simulink model "Funtional_architecture"  (R2023b)
settings: Solver=VariableStepAuto  StartTime=0.0  StopTime=10.0  RelTol=1e-3
settings Model: Creator=Cristian  LastModifiedBy=Cristian

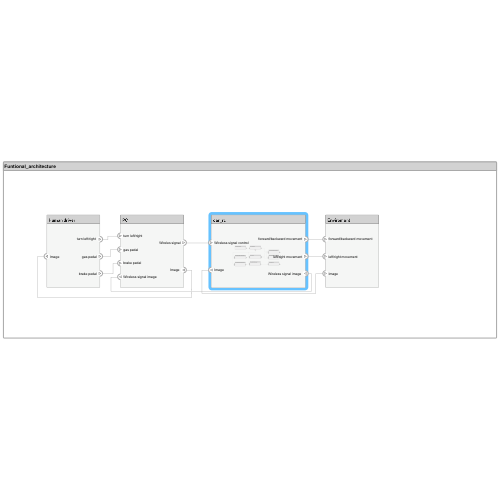
[thumbnail: Simulink's stored preview of the top-level diagram]
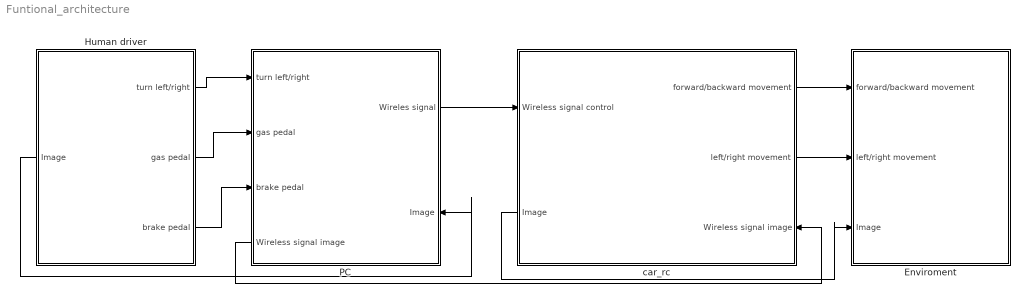
== system Funtional_architecture ==
  Enviroment : Subsystem
      settings: PortSchema="{\"entries\":[{\"content\":{\"headerSize\":26,\"margin\":15,\"minimumSpacing\":25,\"sides\":[{\"content\":{\"connectorIds\":[\"In1\",\"In3\",\"In2\"]},\"type\":\"ConnectorPlacement.EquallySpacedRectSide\",\"uuid\":\"91bad662-27d1-4d59-a5f7-74e6234eecbb\"},{\"content\":{\"side\":\"RIGHT\"},\"type\":\"ConnectorPlacement.EquallySpacedRectSide\",\"uuid\":\"82f07ea1-3832-41bc-8b24-b125feaa4e94\"},{\"content\":{\"side\":\"TOP\"},\"type\":\"ConnectorPlacement.EquallySpacedRectSide\",\"uuid\":\"b3c061be-027d-4d14-becf-7da3730053c6\"}]},\"type\":\"ConnectorPlacement.EquallySpacedConnector\",\"uuid\":\"02efdf8c-4bde-4c3a-95c2-4e1e7b2b6121\"}],\"packageUris\":[\"http://schema.mathworks.com/mf0/Connector/R2020b\"],\"version\":\"1.0\"}"
  Human driver : Subsystem
      settings: PortSchema="{\"entries\":[{\"content\":{\"headerSize\":26,\"margin\":15,\"minimumSpacing\":25,\"sides\":[{\"content\":{\"connectorIds\":[\"Out4\"]},\"type\":\"ConnectorPlacement.EquallySpacedRectSide\",\"uuid\":\"91bad662-27d1-4d59-a5f7-74e6234eecbb\"},{\"content\":{\"connectorIds\":[\"Out1\",\"Out2\",\"Out3\"],\"side\":\"RIGHT\"},\"type\":\"ConnectorPlacement.EquallySpacedRectSide\",\"uuid\":\"82f07ea1-3832-41bc-8b24-b125feaa4e94\"},{\"content\":{\"side\":\"TOP\"},\"type\":\"ConnectorPlacement.EquallySpacedRectSide\",\"uuid\":\"b3c061be-027d-4d14-becf-7da3730053c6\"}]},\"type\":\"ConnectorPlacement.EquallySpacedConnector\",\"uuid\":\"02efdf8c-4bde-4c3a-95c2-4e1e7b2b6121\"}],\"packageUris\":[\"http://schema.mathworks.com/mf0/Connector/R2020b\"],\"version\":\"1.0\"}"
  PC : Subsystem
      settings: PortSchema="{\"entries\":[{\"content\":{\"headerSize\":26,\"margin\":15,\"minimumSpacing\":25,\"sides\":[{\"content\":{\"connectorIds\":[\"In1\",\"In2\",\"In3\",\"Out2\"]},\"type\":\"ConnectorPlacement.EquallySpacedRectSide\",\"uuid\":\"91bad662-27d1-4d59-a5f7-74e6234eecbb\"},{\"content\":{\"connectorIds\":[\"Out1\",\"In4\"],\"side\":\"RIGHT\"},\"type\":\"ConnectorPlacement.EquallySpacedRectSide\",\"uuid\":\"82f07ea1-3832-41bc-8b24-b125feaa4e94\"},{\"content\":{\"side\":\"TOP\"},\"type\":\"ConnectorPlacement.EquallySpacedRectSide\",\"uuid\":\"b3c061be-027d-4d14-becf-7da3730053c6\"}]},\"type\":\"ConnectorPlacement.EquallySpacedConnector\",\"uuid\":\"02efdf8c-4bde-4c3a-95c2-4e1e7b2b6121\"}],\"packageUris\":[\"http://schema.mathworks.com/mf0/Connector/R2020b\"],\"version\":\"1.0\"}"
  car_rc : Subsystem
      settings: PortSchema="{\"entries\":[{\"content\":{\"headerSize\":26,\"margin\":15,\"minimumSpacing\":25,\"sides\":[{\"content\":{\"connectorIds\":[\"In1\",\"Out2\"]},\"type\":\"ConnectorPlacement.EquallySpacedRectSide\",\"uuid\":\"91bad662-27d1-4d59-a5f7-74e6234eecbb\"},{\"content\":{\"connectorIds\":[\"Out1\",\"Out3\",\"In2\"],\"side\":\"RIGHT\"},\"type\":\"ConnectorPlacement.EquallySpacedRectSide\",\"uuid\":\"82f07ea1-3832-41bc-8b24-b125feaa4e94\"},{\"content\":{\"side\":\"TOP\"},\"type\":\"ConnectorPlacement.EquallySpacedRectSide\",\"uuid\":\"b3c061be-027d-4d14-becf-7da3730053c6\"}]},\"type\":\"ConnectorPlacement.EquallySpacedConnector\",\"uuid\":\"02efdf8c-4bde-4c3a-95c2-4e1e7b2b6121\"}],\"packageUris\":[\"http://schema.mathworks.com/mf0/Connector/R2020b\"],\"version\":\"1.0\"}"
  wires:
  PC/2("Wireless signal image ") -> car_rc/2("Wireless signal image ")
  Human driver/4("Image ") -> PC/4("Image ")
  car_rc/2(Image) -> Enviroment/2(Image)
  Human driver/3(brake pedal) -> PC/3(brake pedal)
  PC/1(Wireles signal) -> car_rc/1(Wireless signal control)
  car_rc/3(left/right movement) -> Enviroment/3(left/right movement)
  car_rc/1(forward/backward movement) -> Enviroment/1(forward/backward movement)
  Human driver/1("turn left/right ") -> PC/1("turn left/right ")
  Human driver/2(gas pedal) -> PC/2(gas pedal)

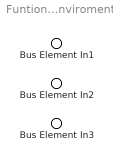
== system Funtional_architecture/Enviroment ==
  Bus Element In1 : Inport  PortName=forward/backward movement
  Bus Element In2 : Inport  Port=2  PortName=Image
  Bus Element In3 : Inport  Port=3  PortName=left/right movement

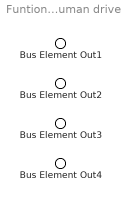
== system Funtional_architecture/Human driver ==
  Bus Element Out1 : Outport  PortName=turn left/right
  Bus Element Out2 : Outport  Port=2  PortName=gas pedal
  Bus Element Out3 : Outport  Port=3  PortName=brake pedal
  Bus Element Out4 : Outport  Port=4  PortName=Image

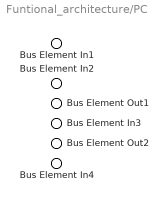
== system Funtional_architecture/PC ==
  Bus Element In1 : Inport  PortName=turn left/right
  Bus Element In2 : Inport  Port=2  PortName=gas pedal
  Bus Element In3 : Inport  Port=3  PortName=brake pedal
  Bus Element In4 : Inport  Port=4  PortName=Image
  Bus Element Out1 : Outport  PortName=Wireles signal
  Bus Element Out2 : Outport  Port=2  PortName=Wireless signal image

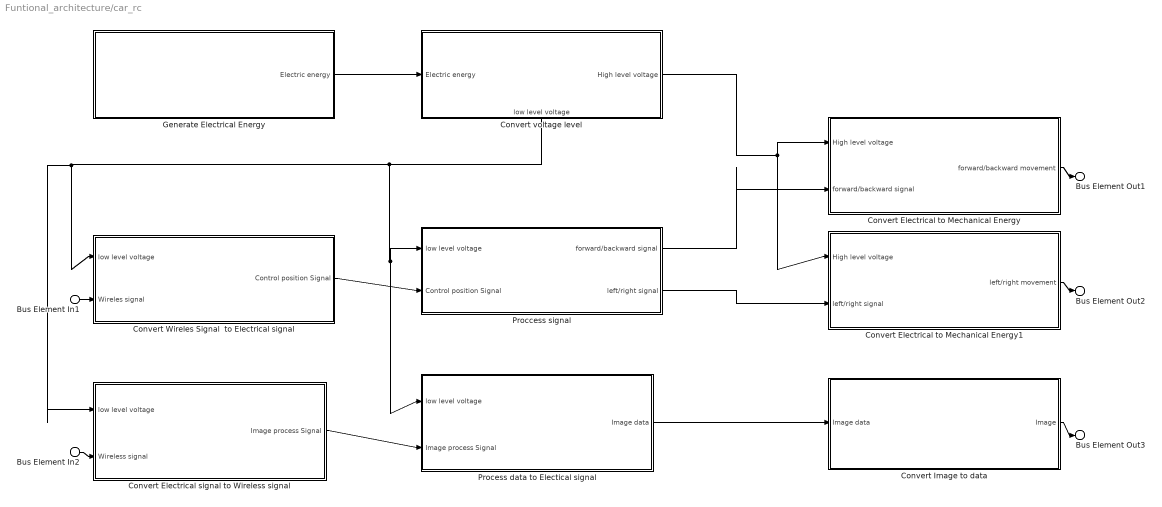
== system Funtional_architecture/car_rc ==
  Bus Element In1 : Inport  PortName=Wireless signal control
  Bus Element In2 : Inport  Port=2  PortName=Wireless signal image
  Convert Electrical signal to Wireless signal : Subsystem
      settings: PortSchema="{\"entries\":[{\"content\":{\"headerSize\":26,\"margin\":15,\"minimumSpacing\":25,\"sides\":[{\"content\":{\"connectorIds\":[\"In1\",\"In2\"]},\"type\":\"ConnectorPlacement.EquallySpacedRectSide\",\"uuid\":\"91bad662-27d1-4d59-a5f7-74e6234eecbb\"},{\"content\":{\"connectorIds\":[\"Out1\"],\"side\":\"RIGHT\"},\"type\":\"ConnectorPlacement.EquallySpacedRectSide\",\"uuid\":\"82f07ea1-3832-41bc-8b24-b125feaa4e94\"},{\"content\":{\"side\":\"TOP\"},\"type\":\"ConnectorPlacement.EquallySpacedRectSide\",\"uuid\":\"b3c061be-027d-4d14-becf-7da3730053c6\"}]},\"type\":\"ConnectorPlacement.EquallySpacedConnector\",\"uuid\":\"02efdf8c-4bde-4c3a-95c2-4e1e7b2b6121\"}],\"packageUris\":[\"http://schema.mathworks.com/mf0/Connector/R2020b\"],\"version\":\"1.0\"}"
  Convert Electrical to Mechanical Energy : Subsystem
      settings: PortSchema="{\"entries\":[{\"content\":{\"headerSize\":26,\"margin\":15,\"minimumSpacing\":25,\"sides\":[{\"content\":{\"connectorIds\":[\"In1\",\"In2\"]},\"type\":\"ConnectorPlacement.EquallySpacedRectSide\",\"uuid\":\"91bad662-27d1-4d59-a5f7-74e6234eecbb\"},{\"content\":{\"connectorIds\":[\"Out1\"],\"side\":\"RIGHT\"},\"type\":\"ConnectorPlacement.EquallySpacedRectSide\",\"uuid\":\"82f07ea1-3832-41bc-8b24-b125feaa4e94\"},{\"content\":{\"side\":\"TOP\"},\"type\":\"ConnectorPlacement.EquallySpacedRectSide\",\"uuid\":\"b3c061be-027d-4d14-becf-7da3730053c6\"}]},\"type\":\"ConnectorPlacement.EquallySpacedConnector\",\"uuid\":\"02efdf8c-4bde-4c3a-95c2-4e1e7b2b6121\"}],\"packageUris\":[\"http://schema.mathworks.com/mf0/Connector/R2020b\"],\"version\":\"1.0\"}"
  Convert Electrical to Mechanical Energy1 : Subsystem
      settings: PortSchema="{\"entries\":[{\"content\":{\"headerSize\":26,\"margin\":15,\"minimumSpacing\":25,\"sides\":[{\"content\":{\"connectorIds\":[\"In1\",\"In2\"]},\"type\":\"ConnectorPlacement.EquallySpacedRectSide\",\"uuid\":\"91bad662-27d1-4d59-a5f7-74e6234eecbb\"},{\"content\":{\"connectorIds\":[\"Out1\"],\"side\":\"RIGHT\"},\"type\":\"ConnectorPlacement.EquallySpacedRectSide\",\"uuid\":\"82f07ea1-3832-41bc-8b24-b125feaa4e94\"},{\"content\":{\"side\":\"TOP\"},\"type\":\"ConnectorPlacement.EquallySpacedRectSide\",\"uuid\":\"b3c061be-027d-4d14-becf-7da3730053c6\"}]},\"type\":\"ConnectorPlacement.EquallySpacedConnector\",\"uuid\":\"02efdf8c-4bde-4c3a-95c2-4e1e7b2b6121\"}],\"packageUris\":[\"http://schema.mathworks.com/mf0/Connector/R2020b\"],\"version\":\"1.0\"}"
  Convert Image to data : Subsystem
      settings: PortSchema="{\"entries\":[{\"content\":{\"headerSize\":26,\"margin\":15,\"minimumSpacing\":25,\"sides\":[{\"content\":{\"connectorIds\":[\"In1\"]},\"type\":\"ConnectorPlacement.EquallySpacedRectSide\",\"uuid\":\"91bad662-27d1-4d59-a5f7-74e6234eecbb\"},{\"content\":{\"connectorIds\":[\"Out1\"],\"side\":\"RIGHT\"},\"type\":\"ConnectorPlacement.EquallySpacedRectSide\",\"uuid\":\"82f07ea1-3832-41bc-8b24-b125feaa4e94\"},{\"content\":{\"side\":\"TOP\"},\"type\":\"ConnectorPlacement.EquallySpacedRectSide\",\"uuid\":\"b3c061be-027d-4d14-becf-7da3730053c6\"}]},\"type\":\"ConnectorPlacement.EquallySpacedConnector\",\"uuid\":\"02efdf8c-4bde-4c3a-95c2-4e1e7b2b6121\"}],\"packageUris\":[\"http://schema.mathworks.com/mf0/Connector/R2020b\"],\"version\":\"1.0\"}"
  Convert Wireles Signal  to Electrical signal : Subsystem
      settings: PortSchema="{\"entries\":[{\"content\":{\"headerSize\":26,\"margin\":15,\"minimumSpacing\":25,\"sides\":[{\"content\":{\"connectorIds\":[\"In1\",\"In2\"]},\"type\":\"ConnectorPlacement.EquallySpacedRectSide\",\"uuid\":\"91bad662-27d1-4d59-a5f7-74e6234eecbb\"},{\"content\":{\"connectorIds\":[\"Out1\"],\"side\":\"RIGHT\"},\"type\":\"ConnectorPlacement.EquallySpacedRectSide\",\"uuid\":\"82f07ea1-3832-41bc-8b24-b125feaa4e94\"},{\"content\":{\"side\":\"TOP\"},\"type\":\"ConnectorPlacement.EquallySpacedRectSide\",\"uuid\":\"b3c061be-027d-4d14-becf-7da3730053c6\"}]},\"type\":\"ConnectorPlacement.EquallySpacedConnector\",\"uuid\":\"02efdf8c-4bde-4c3a-95c2-4e1e7b2b6121\"}],\"packageUris\":[\"http://schema.mathworks.com/mf0/Connector/R2020b\"],\"version\":\"1.0\"}"
  Convert voltage level : Subsystem
      settings: PortSchema="{\"entries\":[{\"content\":{\"headerSize\":26,\"margin\":15,\"minimumSpacing\":25,\"sides\":[{\"content\":{\"connectorIds\":[\"In1\"]},\"type\":\"ConnectorPlacement.EquallySpacedRectSide\",\"uuid\":\"91bad662-27d1-4d59-a5f7-74e6234eecbb\"},{\"content\":{\"connectorIds\":[\"Out1\"],\"side\":\"RIGHT\"},\"type\":\"ConnectorPlacement.EquallySpacedRectSide\",\"uuid\":\"82f07ea1-3832-41bc-8b24-b125feaa4e94\"},{\"content\":{\"side\":\"TOP\"},\"type\":\"ConnectorPlacement.EquallySpacedRectSide\",\"uuid\":\"b3c061be-027d-4d14-becf-7da3730053c6\"},{\"content\":{\"connectorIds\":[\"Out2\"],\"side\":\"BOTTOM\"},\"type\":\"ConnectorPlacement.EquallySpacedRectSide\",\"uuid\":\"1e366329-568c-4f26-bcff-878452f65116\"}]},\"type\":\"ConnectorPlacement.EquallySpacedConnector\",\"uuid\":\"02efdf8c-4bde-4c3a-95c2-4e1e7b2b6121\"}],\"packageUris\":[\"http://schema.mathworks.com/mf0/Connector/R2020b\"],\"version\":\"1.0\"}"
  Generate Electrical Energy : Subsystem
      settings: PortSchema="{\"entries\":[{\"content\":{\"headerSize\":26,\"margin\":15,\"minimumSpacing\":25,\"sides\":[{\"content\":{},\"type\":\"ConnectorPlacement.EquallySpacedRectSide\",\"uuid\":\"91bad662-27d1-4d59-a5f7-74e6234eecbb\"},{\"content\":{\"connectorIds\":[\"Out1\"],\"side\":\"RIGHT\"},\"type\":\"ConnectorPlacement.EquallySpacedRectSide\",\"uuid\":\"82f07ea1-3832-41bc-8b24-b125feaa4e94\"},{\"content\":{\"side\":\"TOP\"},\"type\":\"ConnectorPlacement.EquallySpacedRectSide\",\"uuid\":\"b3c061be-027d-4d14-becf-7da3730053c6\"}]},\"type\":\"ConnectorPlacement.EquallySpacedConnector\",\"uuid\":\"02efdf8c-4bde-4c3a-95c2-4e1e7b2b6121\"}],\"packageUris\":[\"http://schema.mathworks.com/mf0/Connector/R2020b\"],\"version\":\"1.0\"}"
  Proccess signal : Subsystem
      settings: PortSchema="{\"entries\":[{\"content\":{\"headerSize\":26,\"margin\":15,\"minimumSpacing\":25,\"sides\":[{\"content\":{\"connectorIds\":[\"In1\",\"In2\"]},\"type\":\"ConnectorPlacement.EquallySpacedRectSide\",\"uuid\":\"91bad662-27d1-4d59-a5f7-74e6234eecbb\"},{\"content\":{\"connectorIds\":[\"Out1\",\"Out2\"],\"side\":\"RIGHT\"},\"type\":\"ConnectorPlacement.EquallySpacedRectSide\",\"uuid\":\"82f07ea1-3832-41bc-8b24-b125feaa4e94\"},{\"content\":{\"side\":\"TOP\"},\"type\":\"ConnectorPlacement.EquallySpacedRectSide\",\"uuid\":\"b3c061be-027d-4d14-becf-7da3730053c6\"}]},\"type\":\"ConnectorPlacement.EquallySpacedConnector\",\"uuid\":\"02efdf8c-4bde-4c3a-95c2-4e1e7b2b6121\"}],\"packageUris\":[\"http://schema.mathworks.com/mf0/Connector/R2020b\"],\"version\":\"1.0\"}"
  Process data to Electical signal : Subsystem
      settings: PortSchema="{\"entries\":[{\"content\":{\"headerSize\":26,\"margin\":15,\"minimumSpacing\":25,\"sides\":[{\"content\":{\"connectorIds\":[\"In1\",\"In2\"]},\"type\":\"ConnectorPlacement.EquallySpacedRectSide\",\"uuid\":\"91bad662-27d1-4d59-a5f7-74e6234eecbb\"},{\"content\":{\"connectorIds\":[\"Out1\"],\"side\":\"RIGHT\"},\"type\":\"ConnectorPlacement.EquallySpacedRectSide\",\"uuid\":\"82f07ea1-3832-41bc-8b24-b125feaa4e94\"},{\"content\":{\"side\":\"TOP\"},\"type\":\"ConnectorPlacement.EquallySpacedRectSide\",\"uuid\":\"b3c061be-027d-4d14-becf-7da3730053c6\"}]},\"type\":\"ConnectorPlacement.EquallySpacedConnector\",\"uuid\":\"02efdf8c-4bde-4c3a-95c2-4e1e7b2b6121\"}],\"packageUris\":[\"http://schema.mathworks.com/mf0/Connector/R2020b\"],\"version\":\"1.0\"}"
  Bus Element Out1 : Outport  PortName=forward/backward movement
  Bus Element Out3 : Outport  Port=2  PortName=Image
  Bus Element Out2 : Outport  Port=3  PortName=left/right movement
  wires:
  Proccess signal/1(forward/backward signal) -> Convert Electrical to Mechanical Energy/2(forward/backward signal)
  Convert Wireles Signal  to Electrical signal/1(Control position Signal) -> Proccess signal/2(Control position Signal)
  Proccess signal/2(left/right signal) -> Convert Electrical to Mechanical Energy1/2(left/right signal)
  Bus Element In1/1 -> Convert Wireles Signal  to Electrical signal/2(Wireles signal)
  Convert Electrical to Mechanical Energy/1(forward/backward movement) -> Bus Element Out1/1
  Convert Electrical to Mechanical Energy1/1(left/right movement) -> Bus Element Out2/1
  Convert Image to data/1(Image) -> Bus Element Out3/1
  Process data to Electical signal/1(Image data) -> Convert Image to data/1(Image data)
  Convert Electrical signal to Wireless signal/1(Image process Signal) -> Process data to Electical signal/2(Image process Signal)
  Bus Element In2/1 -> Convert Electrical signal to Wireless signal/2("Wireless signal ")
  Generate Electrical Energy/1(Electric energy) -> Convert voltage level/1(Electric energy)
  Convert voltage level/2(low level voltage) -> Convert Electrical signal to Wireless signal/1(low level voltage), Convert Wireles Signal  to Electrical signal/1(low level voltage), Process data to Electical signal/1(low level voltage), Proccess signal/1(low level voltage)
  Convert voltage level/1(High level voltage) -> Convert Electrical to Mechanical Energy1/1(High level voltage), Convert Electrical to Mechanical Energy/1(High level voltage)

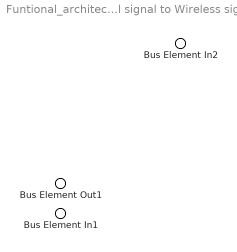
== system Funtional_architecture/car_rc/Convert Electrical signal to Wireless signal ==
  Bus Element In2 : Inport  PortName=low level voltage
  Bus Element In1 : Inport  Port=2  PortName=Wireless signal
  Bus Element Out1 : Outport  PortName=Image process Signal

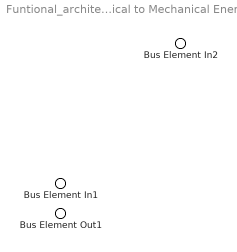
== system Funtional_architecture/car_rc/Convert Electrical to Mechanical Energy ==
  Bus Element In2 : Inport  PortName=High level voltage
  Bus Element In1 : Inport  Port=2  PortName=forward/backward signal
  Bus Element Out1 : Outport  PortName=forward/backward movement

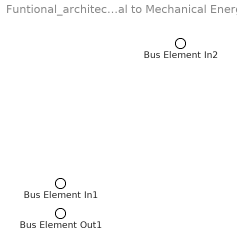
== system Funtional_architecture/car_rc/Convert Electrical to Mechanical Energy1 ==
  Bus Element In2 : Inport  PortName=High level voltage
  Bus Element In1 : Inport  Port=2  PortName=left/right signal
  Bus Element Out1 : Outport  PortName=left/right movement

== system Funtional_architecture/car_rc/Convert Image to data ==
  Bus Element In1 : Inport  PortName=Image data
  Bus Element Out1 : Outport  PortName=Image

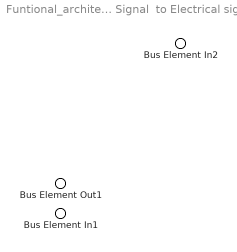
== system Funtional_architecture/car_rc/Convert Wireles Signal  to Electrical signal ==
  Bus Element In2 : Inport  PortName=low level voltage
  Bus Element In1 : Inport  Port=2  PortName=Wireles signal
  Bus Element Out1 : Outport  PortName=Control position Signal

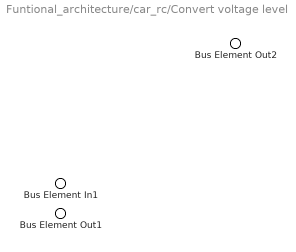
== system Funtional_architecture/car_rc/Convert voltage level ==
  Bus Element In1 : Inport  PortName=Electric energy
  Bus Element Out2 : Outport  PortName=High level voltage
  Bus Element Out1 : Outport  Port=2  PortName=low level voltage

== system Funtional_architecture/car_rc/Generate Electrical Energy ==
  Bus Element Out1 : Outport  PortName=Electric energy

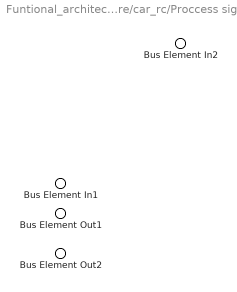
== system Funtional_architecture/car_rc/Proccess signal ==
  Bus Element In2 : Inport  PortName=low level voltage
  Bus Element In1 : Inport  Port=2  PortName=Control position Signal
  Bus Element Out1 : Outport  PortName=forward/backward signal
  Bus Element Out2 : Outport  Port=2  PortName=left/right signal

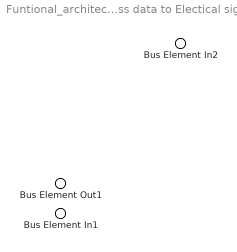
== system Funtional_architecture/car_rc/Process data to Electical signal ==
  Bus Element In2 : Inport  PortName=low level voltage
  Bus Element In1 : Inport  Port=2  PortName=Image process Signal
  Bus Element Out1 : Outport  PortName=Image data
